simulink model "arduino_pi_bt"  (R2013b)
settings: Solver=ode3  SolverMode=SingleTasking  StartTime=0.0  StopTime=inf  FixedStep=1  RelTol=1e-3
libraries: arduinolib x3, simulink x2, dspbuff3 x1
settings Model: ExtModeTrigDuration=2  Creator=mjin  LastModifiedBy=scastro
settings OptimizationCC: OptimizeModelRefInitCode=on  LifeSpan=Inf
settings DebuggingCC: SolverPrmCheckMsg=none  StateNameClashWarn=warning
settings HardwareCC: ProdBitPerInt=16  ProdBitPerPointer=8  ProdIntDivRoundTo=Zero  ProdEndianess=LittleEndian  ProdWordSize=8  ProdHWDeviceType=Atmel->AVR
settings RTWCC: SystemTargetFile=realtime.tlc  GenerateMakefile=off  TemplateMakefile=realtime.tmf  Description=Run on Target Hardware  RTWVerbose=off  ProcessScript=realtime_make_rtw_hook
settings STFCustomTargetCC: TargetLibSuffix=.a  GenerateSampleERTMain=on  ERTCustomFileBanners=on  SupportNonInlinedSFcns=off  SupportVariableSizeSignals=on  MATLABClassNameForMDSCustomization=Simulink.SoftwareTarget.ERTCustomization  GRTInterface=off  SystemTargetFile=realtime.tlc
settings ERTTargetCC: CodeReplacementLibrary=ANSI_C  GenerateSampleERTMain=on  ParMdlRefBuildCompliant=off  CompOptLevelCompliant=off  ConcurrentExecutionCompliant=off  CombineOutputUpdateFcns=off  ERTFirstTimeCompliant=off  SupportContinuousTime=on  SupportVariableSizeSignals=on  ModelStepFunctionPrototypeControlCompliant=off  CPPClassGenCompliant=off  ExtMode=on  ExtModeTransport=3  ExtModeMexFile=ext_serial_win32_comm  ExtModeMexArgs=0 8 115200  InlinedParameterPlacement=NonHierarchical  ERTSrcFileBannerTemplate=realtime_code_template.cgt  ERTHdrFileBannerTemplate=realtime_code_template.cgt  ERTDataSrcFileTemplate=realtime_code_template.cgt  ERTDataHdrFileTemplate=realtime_code_template.cgt  ERTCustomFileTemplate=realtime_file_process.tlc

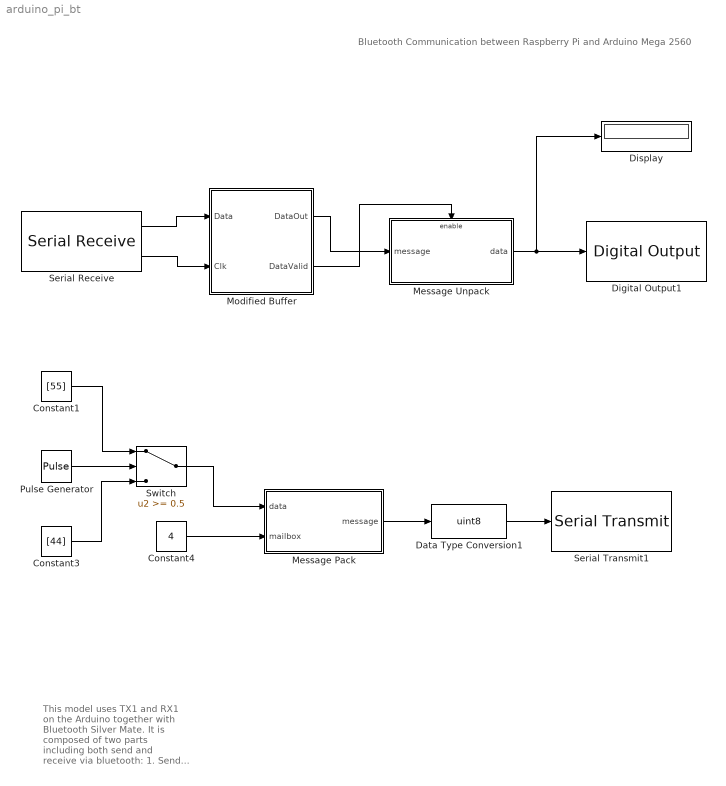
== system arduino_pi_bt ==
  note: This model uses TX1 and RX1 on the Arduino together with Bluetooth Silver Mate. It is composed of two parts including both send and receive via bluetooth:
      | 1. Send (from Arduino to Pi): given data, either vector or scalar, and mailbox number, the model forms a message in the form of [num_data+1, 0, mailbox, data]
      |  and then sends it out to the COM port, which connects to the Silver Mate and gets transmitted to Pi over bluetooth.
      | 2. Receive (from Pi to Arduino): given expected incoming message of length fixed to 4 and in the form of [2, 0, mailbox, scalar_data], the model buffers the data
      | using a counting buffer which triggers the unpack subsystem whenever the buffer is full. At last, it extracts the data element.
      |
      | NOTE: Change the COM port in Config Params to either Automatic or the proper one for your Arduino board before running it.
  note: Bluetooth Communication between Raspberry Pi and Arduino Mega 2560
  Constant1 : Constant  Value=[55]
  Constant3 : Constant  Value=[44]
  Constant4 : Constant  Value=4
  Data Type Conversion1 : DataTypeConversion  OutDataTypeStr=uint8
  Digital Output1 : arduinolib/Digital Output  pinNumber=13
  Display : Display
  Message Pack : Subsystem
  Message Unpack : Subsystem  TreatAsAtomicUnit=on
  Modified Buffer : Subsystem  TreatAsAtomicUnit=on  mask(Input-Driven Buffer){bufSize=4}
      mask prompts: bufSize "Buffer size:"
      mask help: A modified buffer subsystem that is driven by the arrival of its input data; it produces a valid output data buffer whenever its buffer is full and sets its dataValid flag to 1. Otherwise, the data at its dataOut port is not valid and its dataValid flag is set to 0.
      settings: AttributesFormatString=Counting Buffer
      mask Display: disp('Modified Buffer')
  Pulse Generator : DiscretePulseGenerator  PulseType=Time based  Period=4  PulseWidth=50
  Serial Receive : arduinolib/Serial Receive  portNumber=1  showOutStatus=on  sampleTime=1
  Serial Transmit1 : arduinolib/Serial Transmit  portNumber=1
  Switch : Switch  Threshold=0.5
  wires:
  Constant4/1 -> Message Pack/2(mailbox)
  Message Pack/1(message) -> Data Type Conversion1/1
  Constant1/1 -> Switch/1
  Constant3/1 -> Switch/3
  Pulse Generator/1 -> Switch/2
  Data Type Conversion1/1 -> Serial Transmit1/1
  Switch/1 -> Message Pack/1(data)
  Message Unpack/1(data) -> Display/1, Digital Output1/1
  Serial Receive/1 -> Modified Buffer/1(Data)
  Serial Receive/2 -> Modified Buffer/2(Clk)
  Modified Buffer/2(DataValid) -> Message Unpack/Enable
  Modified Buffer/1(DataOut) -> Message Unpack/1(message)

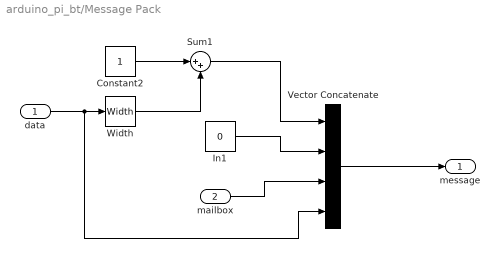
== system arduino_pi_bt/Message Pack ==
  data : Inport
  mailbox : Inport  Port=2
  Constant2 : Constant
  In1 : Constant  Value=0
  Sum1 : Sum  Inputs=|++
  Vector Concatenate : Concatenate  NumInputs=4
  Width : Width
  message : Outport
  wires:
  Constant2/1 -> Sum1/1
  In1/1 -> Vector Concatenate/2
  data/1 -> Vector Concatenate/4, Width/1
  Vector Concatenate/1 -> message/1
  mailbox/1 -> Vector Concatenate/3
  Sum1/1 -> Vector Concatenate/1
  Width/1 -> Sum1/2

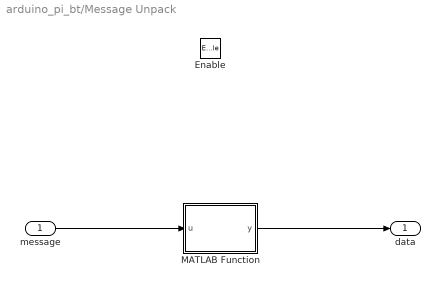
== system arduino_pi_bt/Message Unpack ==
  message : Inport
  Enable : EnablePort
  MATLAB Function : MATLAB Function  TreatAsAtomicUnit=on
  data : Outport
  wires:
  message/1 -> MATLAB Function/1(u)
  MATLAB Function/1(y) -> data/1

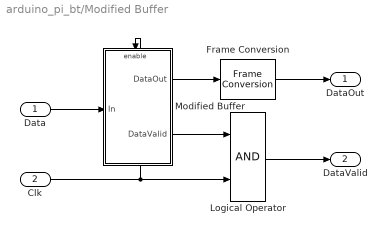
== system arduino_pi_bt/Modified Buffer ==
  Data : Inport
  Clk : Inport  Port=2
  Frame Conversion : FrameConversion  OutFrame=Sample-based
  Logical Operator : Logic  AllPortsSameDT=off  OutDataTypeStr=boolean
  Modified Buffer : Subsystem
  DataOut : Outport
  DataValid : Outport  Port=2
  wires:
  Clk/1 -> Logical Operator/2, Modified Buffer/Enable
  Frame Conversion/1 -> DataOut/1
  Logical Operator/1 -> DataValid/1
  Modified Buffer/2(DataValid) -> Logical Operator/1
  Modified Buffer/1(DataOut) -> Frame Conversion/1
  Data/1 -> Modified Buffer/1(In)

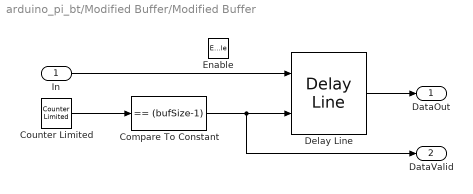
== system arduino_pi_bt/Modified Buffer/Modified Buffer ==
  In : Inport
  Enable : EnablePort
  Compare To Constant : simulink/Logic and Bit Operations/Compare To Constant  relop===  const=(bufSize-1)  OutDataTypeStr=boolean  ZeroCross=off
  Counter Limited : simulink/Sources/Counter Limited  uplimit=(bufSize-1)  tsamp=-1
  Delay Line : dspbuff3/Delay Line  siz=bufSize  ic=0  directfeed=on  enable_output=on  hold_output=off  TreatMby1Signals=One channel
  DataOut : Outport
  DataValid : Outport  Port=2
  wires:
  Counter Limited/1 -> Compare To Constant/1
  In/1 -> Delay Line/1
  Delay Line/1 -> DataOut/1
  Compare To Constant/1 -> DataValid/1, Delay Line/2

== matlab function arduino_pi_bt/Message Unpack/MATLAB Function ==
  data: u input; y output
function y = fcn(u)
%#codegen

zero_index = find(u==0);
if zero_index(1)+2<=4
    value_index = zero_index(1)+2;
else
    value_index = mod((zero_index(1)+2),4);
end
y = u(value_index);
